simulink model "sim_arcfault"  (R2014a)
settings: Solver=ode14x  StartTime=0.0  StopTime=80e-3  FixedStep=1e-6  RelTol=1e-5
libraries: fl_lib x4, nesl_utility x4, elec_lib x1, ArcLib_lib x1
settings Model: Creator=Dr J  LastModifiedBy=Dr J

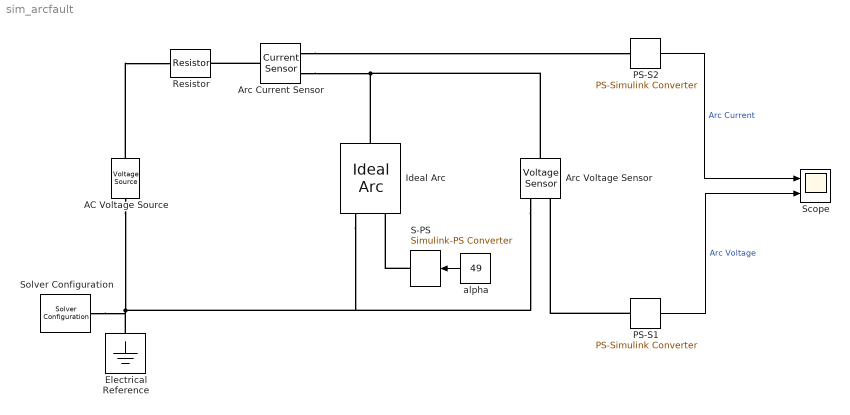
== system sim_arcfault ==
  AC Voltage Source : elec_lib/Sources/Voltage Source  dc_voltage=0 V  ac_voltage=200 V  ac_shift=0 deg  ac_frequency=50 Hz  noise_mode=0  PSD=0 V^2/Hz  sample_time=0.001 s  repeatability=1  auto_seed=3499211588  user_seed=0
  Arc Current Sensor : fl_lib/Electrical/Electrical Sensors/Current Sensor
  Arc Voltage Sensor : fl_lib/Electrical/Electrical Sensors/Voltage Sensor
  Electrical Reference : fl_lib/Electrical/Electrical Elements/Electrical Reference
  Ideal Arc : ArcLib_lib/Ideal Arc  b=1.46  Rc=2221 Ohm  TauV=0.0001 s  TauI=0.00001 s  i_specify=on  i_priority=High  i=0.001 A  v_specify=on  v_priority=High  v=0.001 V  it_specify=on  it_priority=High  it=1e-4 A
  PS-S1 : nesl_utility/PS-Simulink Converter  PhysicalDomain=network_engine_domain  SubClassName=ps_output  LeftPortType=input  RightPortType=output  PseudoPeriodic=off  Frequencies=[]  Unit=1  AffineConversion=off
  PS-S2 : nesl_utility/PS-Simulink Converter  PhysicalDomain=network_engine_domain  SubClassName=ps_output  LeftPortType=input  RightPortType=output  PseudoPeriodic=off  Frequencies=[]  Unit=1  AffineConversion=off
  Resistor : fl_lib/Electrical/Electrical Elements/Resistor  R=43 Ohm  i_specify=off  i_priority=High  i=10 A  v_specify=off  v_priority=High  v=0 V
  S-PS : nesl_utility/Simulink-PS Converter  PhysicalDomain=network_engine_domain  SubClassName=ps_input  LeftPortType=input  RightPortType=output  PseudoPeriodic=off  Frequencies=[]  NoiseDistribution=none  NoiseParameters=[]  Unit=1  AffineConversion=off  InputFiltering=off  SimscapeFilterOrder=1  InputFilterTimeConstant=0.001  UdotUserProvided=1
  Scope : Scope  NumInputPorts=2
      settings: YMin=-4~-150  YMax=4~150
  Solver Configuration : nesl_utility/Solver Configuration  PhysicalDomain=network_engine_domain  SubClassName=solver  LeftPortType=input  RightPortType=generic  Accelerate=off  Tones=[]  Harmonics=[]  SimulateNoise=off  Profile=off  UseLocalSampling=off  EnableSwitchedLinearOptims=on  FrequencyDomain=off  UseCCode=off  RelTol=0.001  AbsTol=1e-06  MinStep=1e-09  ToWorkspace=off  DoDC=off  ResidualTolerance=1e-09  UseLocalSolver=on  LocalSolverChoice=NE_BACKWARD_EULER_ADVANCER  LocalSolverSampleTime=1e-6  DoFixedCost=on  MaxNonlinIter=3  MaxModeIter=2  LinearAlgebra=Sparse  DelaysMemoryBudget=1024  AutomaticFiltering=on  FilteringTimeConstant=0.001
  alpha : Constant  Value=49
  wires:
  alpha/1 -> S-PS/1
  PS-S2/1 -> Scope/1  "Arc Current"
  PS-S1/1 -> Scope/2  "Arc Voltage"
  connections:
  AC Voltage Source/LConn1 -- Resistor/LConn1
  AC Voltage Source/RConn1 -- Solver Configuration/RConn1 -- Electrical Reference/LConn1 -- Arc Voltage Sensor/RConn2 -- Ideal Arc/RConn1
  Arc Voltage Sensor/LConn1 -- Arc Current Sensor/RConn2 -- Ideal Arc/LConn1
  PS-S1/LConn1 -- Arc Voltage Sensor/RConn1
  Arc Current Sensor/LConn1 -- Resistor/RConn1
  Arc Current Sensor/RConn1 -- PS-S2/LConn1
  S-PS/RConn1 -- Ideal Arc/RConn2
